simulink model "sine_decay_colornoise"  (R2017a)
settings: Solver=VariableStepAuto  StartTime=0.0  StopTime=10.0  RelTol=1e-3
libraries: simulink x1, dspsrcs4 x1
settings Model: Creator=ljxia  LastModifiedBy=ljxia

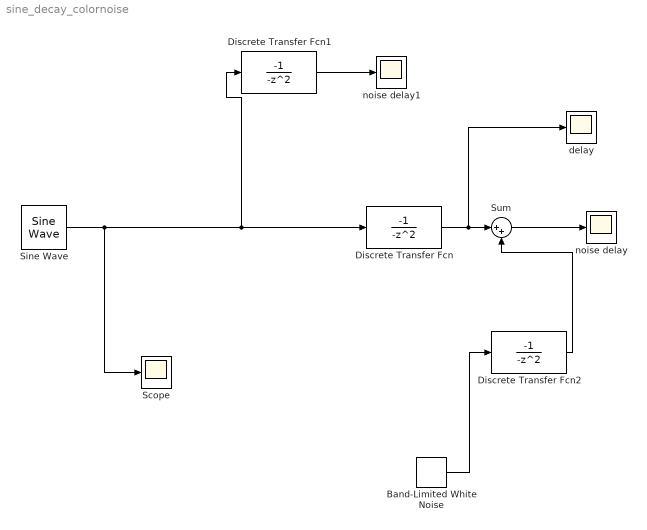
== system sine_decay_colornoise ==
  Band-Limited White Noise : simulink/Sources/Band-Limited White Noise  Cov=[1]  Ts=0.01  seed=[23342]
  Discrete Transfer Fcn : DiscreteTransferFcn  Numerator=[-1]  Denominator=[-1 0 0]
  Discrete Transfer Fcn1 : DiscreteTransferFcn  Numerator=[-1]  Denominator=[-1 0 0]
  Discrete Transfer Fcn2 : DiscreteTransferFcn  Numerator=[-1]  Denominator=[-1 0 0]
  Scope : Scope
  Sine Wave : dspsrcs4/Sine Wave  Amplitude=1  Frequency=10  Phase=0  SampleMode=Discrete  OutComplex=Real  CompMethod=Trigonometric fcn  TableSize=Speed  SampleTime=1/100  SamplesPerFrame=1  ResetState=Restart at time zero  OutputFrames=off  dataType=double  wordLen=16  udDataType=sfix(16)  fracBitsMode=Best precision  numFracBits=15  OutDataTypeStr=double  LastOutDataTypeStr=double
  Sum : Sum  Inputs=|++
  delay : Scope
  noise delay : Scope
  noise delay1 : Scope
  wires:
  Discrete Transfer Fcn1/1 -> noise delay1/1
  Sine Wave/1 -> Discrete Transfer Fcn/1, Discrete Transfer Fcn1/1, Scope/1
  Sum/1 -> noise delay/1
  Discrete Transfer Fcn/1 -> delay/1, Sum/1
  Band-Limited White Noise/1 -> Discrete Transfer Fcn2/1
  Discrete Transfer Fcn2/1 -> Sum/2
